simulink model "Manual_Control"  (R2020a)
settings: Solver=FixedStepAuto  StartTime=0.0  StopTime=inf  RelTol=1e-3
model workspace (MAT data in the model file):
  SL_ROS_VariableLengthArrays_MaxSizes.CommonInfo.ArrayTruncateAction = 'EmitWarning'
  SL_ROS_VariableLengthArrays_MaxSizes.MsgTypeMap = containers.Map
  SL_ROS_VariableLengthArrays_MaxSizes.MsgTypeMap.serialization.keys = {'sensor_msgs/LaserScan'}
  SL_ROS_VariableLengthArrays_MaxSizes.MsgTypeMap.serialization.values{1}(1).PropertyName = 'Intensities'
  SL_ROS_VariableLengthArrays_MaxSizes.MsgTypeMap.serialization.values{1}(1).DataType = 'single'
  SL_ROS_VariableLengthArrays_MaxSizes.MsgTypeMap.serialization.values{1}(1).MaxLength = 360
  SL_ROS_VariableLengthArrays_MaxSizes.MsgTypeMap.serialization.values{1}(2).PropertyName = 'Ranges'
  SL_ROS_VariableLengthArrays_MaxSizes.MsgTypeMap.serialization.values{1}(2).DataType = 'single'
  SL_ROS_VariableLengthArrays_MaxSizes.MsgTypeMap.serialization.values{1}(2).MaxLength = 360
  SL_ROS_VariableLengthArrays_MaxSizes.MsgTypeMap.serialization.uniformity = 0
  SL_ROS_VariableLengthArrays_MaxSizes.MsgTypeMap.serialization.keyType = 'char'
  SL_ROS_VariableLengthArrays_MaxSizes.MsgTypeMap.serialization.valueType = 'any'
undefined symbols (not defined in the file): Angular, Linear
libraries: robotlib x2, realtime_pacer_lib x2, simulink_extras x1, vrlib x1
settings Model: Creator=20195009  LastModifiedBy=TruckLabPC2
settings OptimizationCC: EnhancedBackFolding=on  PassReuseOutputArgsAs=Individual arguments  ZeroExternalMemoryAtStartup=off  ZeroInternalMemoryAtStartup=off  MaxStackSize=64  OptimizeBlockOrder=speed  DifferentSizesBufferReuse=on  OptimizationCustomize=off  EfficientTunableParamExpr=on
settings DebuggingCC: ParameterTunabilityLossMsg=error  SFMachineParentedDataDiag=error
settings HardwareCC: ProdBitPerPointer=32  ProdBitPerSizeT=32  ProdBitPerPtrDiffT=32  ProdLargestAtomicFloat=None  ProdIntDivRoundTo=Undefined  ProdEndianess=Unspecified  ProdWordSize=32  ProdHWDeviceType=Generic->Unspecified (assume 32-bit Generic)
settings SFSimCC: MATLABDynamicMemAlloc=off
settings RTWCC: SystemTargetFile=ert.tlc  HardwareBoard=Robot Operating System (ROS)  TemplateMakefile=ert_default_tmf  Toolchain=Catkin  TargetLang=C++
settings CodeAppCC: ForceParamTrailComments=on  IgnoreCustomStorageClasses=off  OperatorAnnotations=on  SimulinkDataObjDesc=on  SFDataObjDesc=on  InsertBlockDesc=on

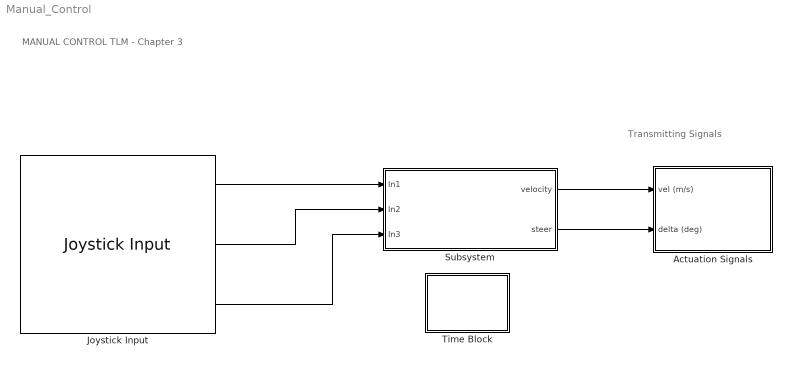
== system Manual_Control ==
  note: MANUAL CONTROL
      | TLM - Chapter 3
  note: Transmitting Signals
  Actuation Signals : Subsystem
  Joystick Input : vrlib/Joystick Input  joyid=1  adjustports=on  forcefeed=off
  Subsystem : Subsystem
  Time Block : Subsystem
  wires:
  Joystick Input/3 -> Subsystem/3(In3)
  Joystick Input/2 -> Subsystem/2(In2)
  Joystick Input/1 -> Subsystem/1(In1)
  Subsystem/2(steer) -> Actuation Signals/2(delta (deg))
  Subsystem/1(velocity) -> Actuation Signals/1(vel (m/s))

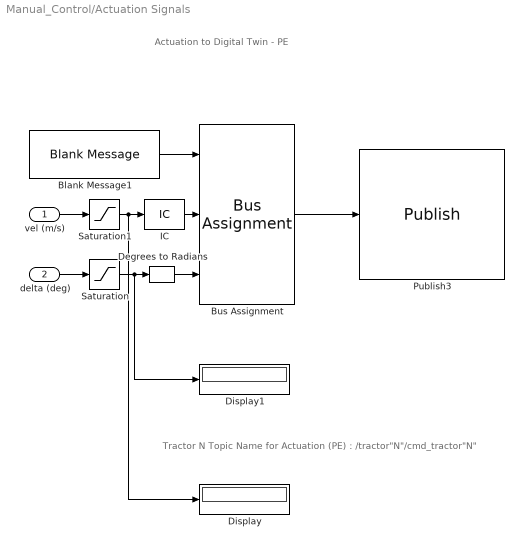
== system Manual_Control/Actuation Signals ==
  note: Tractor N Topic Name for Actuation (PE) : /tractor"N"/cmd_tractor"N"
  note: Actuation to Digital Twin - PE
  vel (m/s) : Inport
  delta (deg) : Inport  Port=2
  Blank Message1 : robotlib/Blank Message  messageClass=Message  entityType=geometry_msgs/Twist  messageType=geometry_msgs/Twist  SampleTime=0.01  legacyBusStruct=off
  Bus Assignment : BusAssignment  DialogController=Simulink.DDGSource_BusAssignment  AssignedSignals=Linear.X,Angular.Z
  Degrees to Radians : simulink_extras/Transformations/Degrees to Radians
  Display : Display
  Display1 : Display
  IC : InitialCondition  Value=0
  Publish3 : robotlib/Publish  topicSource=Select from ROS network  topic=/tractor1/cmd_tractor1  messageType=geometry_msgs/Twist  legacyBusStruct=off  messageQueueLength=1
      link override SinkBlock: ROSTopic=/cmd_vel  ROSMessageType=geometry_msgs/Twist  SLBusName=SL_Bus_TruckLab_MannualDrivingROS1_geometry_msgs_Twist  ModelName=TruckLab_MannualDrivingROS1  BlockId=Pub_TruckLab_MannualDrivingROS1_402
  Saturation : Saturate  UpperLimit=25  LowerLimit=-25
  Saturation1 : Saturate  UpperLimit=0.28  LowerLimit=-0.28
  wires:
  vel (m/s)/1 -> Saturation1/1
  IC/1 -> Bus Assignment/2
  Bus Assignment/1 -> Publish3/1
  Degrees to Radians/1 -> Bus Assignment/3
  Blank Message1/1 -> Bus Assignment/1
  delta (deg)/1 -> Saturation/1
  Saturation/1 -> Display1/1, Degrees to Radians/1
  Saturation1/1 -> Display/1, IC/1

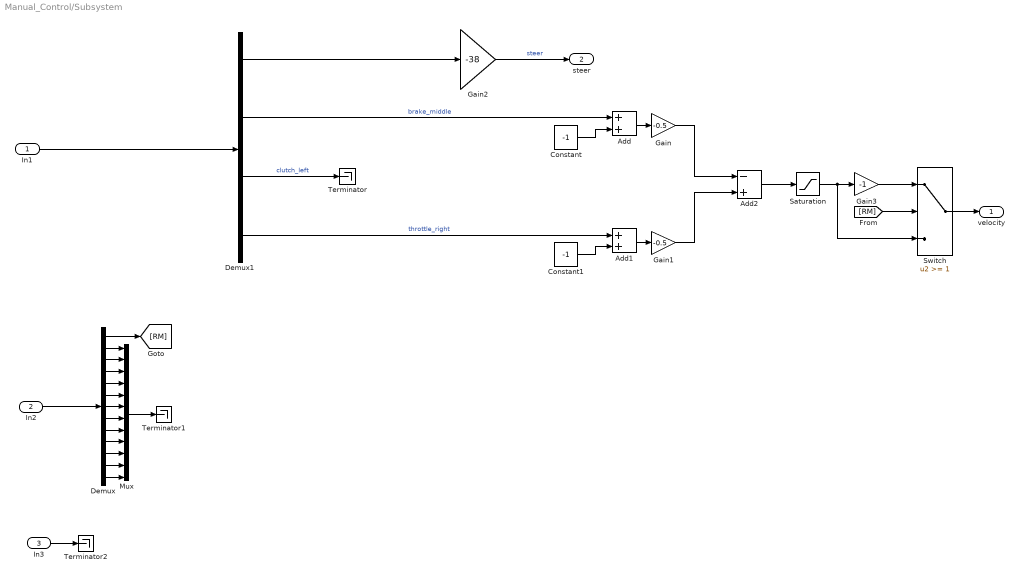
== system Manual_Control/Subsystem ==
  In1 : Inport
  In2 : Inport  Port=2
  In3 : Inport  Port=3
  Add : Sum
  Add1 : Sum
  Add2 : Sum  Inputs=-+
  Constant : Constant  Value=-1
  Constant1 : Constant  Value=-1
  Demux : Demux  Outputs=13
  Demux1 : Demux
  Gain : Gain  Gain=-0.5
  Gain1 : Gain  Gain=-0.5
  Gain2 : Gain  Gain=-38
  Gain3 : Gain  Gain=-1
  Mux : Mux  Inputs=12
  Saturation : Saturate  UpperLimit=5  LowerLimit=0
  Switch : Switch  Threshold=1
  Terminator : Terminator
  Terminator1 : Terminator
  Terminator2 : Terminator
  velocity : Outport
  steer : Outport  Port=2
  wires:
  [RM] -> Switch/2
  Gain3/1 -> Switch/1
  Demux1/4 -> Add1/1  "throttle_right"
  Switch/1 -> velocity/1
  Demux/1 -> [RM]
  Demux1/3 -> Terminator/1  "clutch_left"
  Mux/1 -> Terminator1/1
  In1/1 -> Demux1/1
  In2/1 -> Demux/1
  Demux/6 -> Mux/5
  Demux1/1 -> Gain2/1
  Demux/8 -> Mux/7
  In3/1 -> Terminator2/1
  Constant1/1 -> Add1/2
  Constant/1 -> Add/2
  Demux/9 -> Mux/8
  Demux/12 -> Mux/11
  Demux/5 -> Mux/4
  Demux/3 -> Mux/2
  Demux/10 -> Mux/9
  Gain2/1 -> steer/1  "steer"
  Gain1/1 -> Add2/2
  Add/1 -> Gain/1
  Demux1/2 -> Add/1  "brake_middle"
  Add2/1 -> Saturation/1
  Demux/7 -> Mux/6
  Demux/11 -> Mux/10
  Saturation/1 -> Switch/3, Gain3/1
  Demux/2 -> Mux/1
  Add1/1 -> Gain1/1
  Gain/1 -> Add2/1
  Demux/13 -> Mux/12
  Demux/4 -> Mux/3

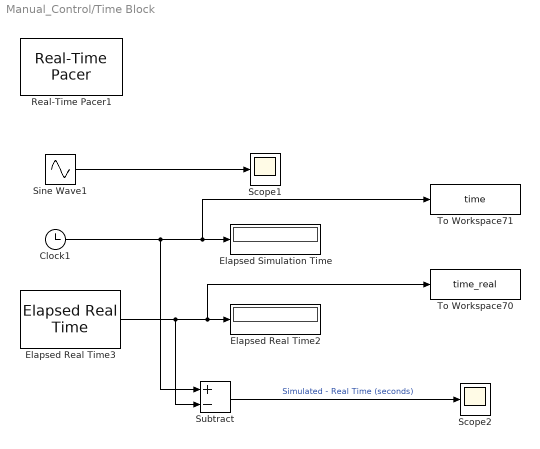
== system Manual_Control/Time Block ==
  Clock1 : Clock
  Elapsed Real Time2 : Display
      settings: Decimation=2
  Elapsed Real Time3 : realtime_pacer_lib/Elapsed Real Time
  Elapsed Simulation Time : Display
      settings: Decimation=2
  Real-Time Pacer1 : realtime_pacer_lib/Real-Time Pacer  simTimePerRealTime=1
  Scope1 : Scope
  Scope2 : Scope
  Sine Wave1 : Sin  Frequency=2*pi*0.5  SampleTime=0
  Subtract : Sum  Inputs=+-
  To Workspace70 : ToWorkspace  VariableName=time_real  SampleTime=-1
  To Workspace71 : ToWorkspace  VariableName=time  SampleTime=-1
  wires:
  Subtract/1 -> Scope2/1  "Simulated - Real Time (seconds)"
  Elapsed Real Time3/1 -> Elapsed Real Time2/1, To Workspace70/1, Subtract/2
  Sine Wave1/1 -> Scope1/1
  Clock1/1 -> Subtract/1, Elapsed Simulation Time/1, To Workspace71/1
